simulink model "Ki_Effect"  (R2024b)
settings: Solver=FixedStepAuto  StartTime=0.0  StopTime=60  FixedStep=1e-3  RelTol=1e-3
settings Model: Creator=abdal  LastModifiedBy=abdal

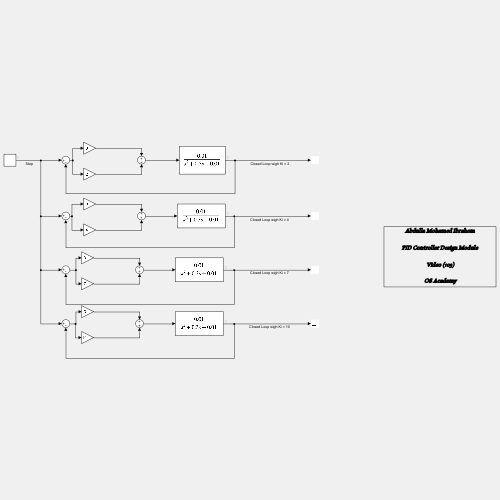
[thumbnail: Simulink's stored preview of the top-level diagram]
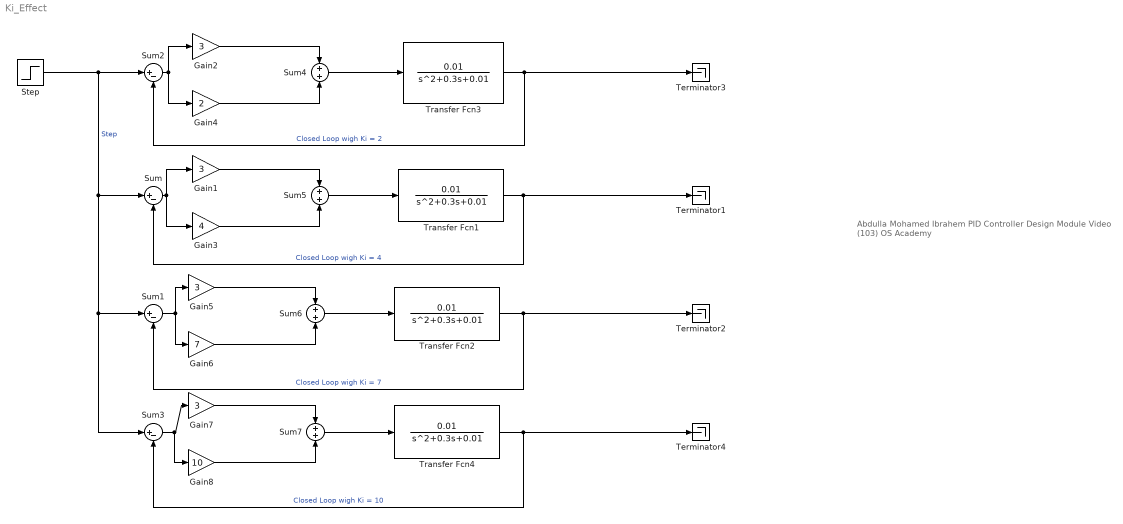
== system Ki_Effect ==
  note: Abdulla Mohamed Ibrahem
      | PID Controller Design Module
      | Video (103)
      | OS Academy
  Gain{1..2,5,7} (4 alike) : Gain  Gain=3
  Gain3 : Gain  Gain=4
  Gain4 : Gain  Gain=2
  Gain6 : Gain  Gain=7
  Gain8 : Gain  Gain=10
  Step : Step  SampleTime=0
  Sum{,1..3} (4 alike) : Sum  Inputs=|+-
  Sum{4..7} (4 alike) : Sum
  Terminator{1..4} (4 alike) : Terminator
  Transfer Fcn{1..4} (4 alike) : TransferFcn  Numerator=0.01  Denominator=[1 0.3 0.01]
  wires:
  Transfer Fcn3/1 -> Terminator3/1, Sum2/2  "Closed Loop wigh Ki = 2"
  Transfer Fcn4/1 -> Sum3/2, Terminator4/1  "Closed Loop wigh Ki = 10"
  Transfer Fcn2/1 -> Terminator2/1, Sum1/2  "Closed Loop wigh Ki = 7"
  Step/1 -> Sum2/1, Sum3/1, Sum1/1, Sum/1  "Step"
  Sum2/1 -> Gain4/1, Gain2/1
  Transfer Fcn1/1 -> Terminator1/1, Sum/2  "Closed Loop wigh Ki = 4"
  Gain2/1 -> Sum4/1
  Gain4/1 -> Sum4/2
  Sum4/1 -> Transfer Fcn3/1
  Gain3/1 -> Sum5/2
  Sum/1 -> Gain3/1, Gain1/1
  Sum5/1 -> Transfer Fcn1/1
  Gain1/1 -> Sum5/1
  Gain6/1 -> Sum6/2
  Sum6/1 -> Transfer Fcn2/1
  Sum1/1 -> Gain5/1, Gain6/1
  Gain5/1 -> Sum6/1
  Gain8/1 -> Sum7/2
  Sum7/1 -> Transfer Fcn4/1
  Gain7/1 -> Sum7/1
  Sum3/1 -> Gain8/1, Gain7/1
